simulink model "LQR2"  (R2020a)
settings: Solver=VariableStepAuto  StartTime=0.0  StopTime=15  RelTol=1e-3
values from neighbouring files (symbols this model uses):
  A = zeros(n_states)    [RIP.m]
  B = zeros(n_states,n_inputs)    [RIP.m]
  C = zeros(n_outputs, n_states)    [RIP.m]
  D = zeros(n_outputs, n_inputs)    [RIP.m]
  Ki = K_d_Int(:,1)    [RIP.m]
  Ks = K_d_Int(:,2:end)    [RIP.m]
  Ts = 1/200    (= 0.005)    [RIP.m]
  wc = 2*pi*fc    (= 9.42477796077)    [RIP.m]
libraries: simulink x2
settings Model: Creator=user  LastModifiedBy=user

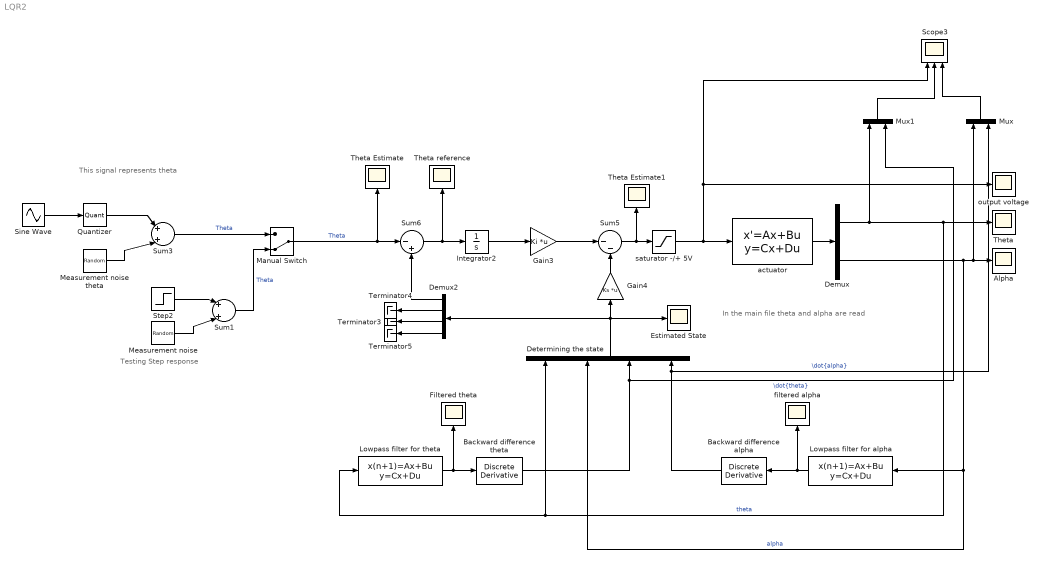
== system LQR2 ==
  note: Testing Step response
  note: This signal represents theta
  note: In the main file theta and alpha are read
  Alpha : Scope
  Backward difference alpha : simulink/Quick Insert/Discrete/Discrete Derivative  gainval=1.0  ICPrevScaledInput=0.0  OutMin=[]  OutMax=[]  OutDataType=fixdt(1, 16)  OutScaling=2^-10  DoSatur=off
      settings: SourceProductBaseCode=SL
  Backward difference theta : simulink/Quick Insert/Discrete/Discrete Derivative  gainval=1.0  ICPrevScaledInput=0.0  OutMin=[]  OutMax=[]  OutDataType=fixdt(1, 16)  OutScaling=2^-10  DoSatur=off
      settings: SourceProductBaseCode=SL
  Demux : Demux  Outputs=2
  Demux2 : Demux
  Determining the state : Mux
  Estimated State : Scope
  Filtered theta : Scope
  Gain3 : Gain  Gain=Ki  Multiplication=Matrix(K*u)
  Gain4 : Gain  Gain=Ks  Multiplication=Matrix(K*u)
  Integrator2 : Integrator
  Lowpass filter for alpha : DiscreteStateSpace  A=1/(1 + wc*Ts)  B=wc*Ts/(1 + wc*Ts)  D=0  SampleTime=Ts
  Lowpass filter for theta : DiscreteStateSpace  A=1/(1 + wc*Ts)  B=wc*Ts/(1 + wc*Ts)  D=0  SampleTime=Ts
  Manual Switch : ManualSwitch  CurrentSetting=0
  Measurement noise : RandomNumber  Variance=0.001  SampleTime=Ts
  Measurement noise theta : RandomNumber  Variance=0.001  SampleTime=Ts
  Mux : Mux  Inputs=2
  Mux1 : Mux  Inputs=2
  Quantizer : Quantizer  QuantizationInterval=pi*2^(-16)
  Scope3 : Scope  NumInputPorts=3
  Sine Wave : Sin  Amplitude=pi/3  Frequency=0.1  SampleTime=Ts
  Step2 : Step  After=pi/3  SampleTime=0
  Sum1 : Sum  Inputs=|+|+|
  Sum3 : Sum  Inputs=|+|+|
  Sum5 : Sum  Inputs=|--
  Sum6 : Sum  Inputs=|-+
  Terminator3 : Terminator
  Terminator4 : Terminator
  Terminator5 : Terminator
  Theta : Scope
  Theta Estimate : Scope
  Theta Estimate1 : Scope
  Theta reference : Scope
  actuator : StateSpace  A=A  B=B  C=C  D=D  InitialCondition=0
  filtered alpha : Scope
  output voltage : Scope
  saturator -/+ 5V : Saturate  UpperLimit=5  LowerLimit=-5
  wires:
  Manual Switch/1 -> Sum6/1, Theta Estimate/1  "Theta"
  Integrator2/1 -> Gain3/1
  Gain4/1 -> Sum5/2
  Measurement noise theta/1 -> Sum3/2
  Demux2/3 -> Terminator3/1
  Quantizer/1 -> Sum3/1
  Demux2/2 -> Terminator4/1
  Gain3/1 -> Sum5/1
  actuator/1 -> Demux/1
  Sum6/1 -> Theta reference/1, Integrator2/1
  Demux2/4 -> Terminator5/1
  Demux2/1 -> Sum6/2
  Lowpass filter for alpha/1 -> Backward difference alpha/1, filtered alpha/1
  Lowpass filter for theta/1 -> Backward difference theta/1, Filtered theta/1
  Determining the state/1 -> Demux2/1, Gain4/1, Estimated State/1
  Backward difference theta/1 -> Mux1/2, Determining the state/3  "\\dot{theta}"
  Backward difference alpha/1 -> Mux/2, Determining the state/4  "\\dot{alpha}"
  Sine Wave/1 -> Quantizer/1
  Sum5/1 -> Theta Estimate1/1, saturator -/+ 5V/1
  Demux/2 -> Alpha/1, Mux/1, Determining the state/2, Lowpass filter for alpha/1  "alpha"
  Demux/1 -> Mux1/1, Lowpass filter for theta/1, Determining the state/1, Theta/1  "theta"
  Sum3/1 -> Manual Switch/1  "Theta"
  Step2/1 -> Sum1/1
  Measurement noise/1 -> Sum1/2
  Sum1/1 -> Manual Switch/2  "Theta"
  saturator -/+ 5V/1 -> actuator/1, Scope3/1, output voltage/1
  Mux/1 -> Scope3/3
  Mux1/1 -> Scope3/2
